simulink model "soc_WLAN_fpga"  (R2024b)
settings: Solver=FixedStepDiscrete  StartTime=0.0  StopTime=stopTime  RelTol=1e-3
PreLoadFcn:
  | addpath(fullfile(matlabroot,'toolbox','whdl','whdlexamples','whdlexamples'));
InitFcn:
  | addpath(fullfile(matlabroot,'toolbox','whdl','whdlexamples','whdlexamples'));
model workspace (MAT data in the model file):
  socvcb = containers.Map
  socvcb.serialization.keys = {}
  socvcb.serialization.values = {}
  socvcb.serialization.uniformity = 0
  socvcb.serialization.keyType = 'double'
  socvcb.serialization.valueType = 'any'
undefined symbols (not defined in the file): Add, bitRatePerOfdmSym, chanBW, coe, cpLen, dataUpsampleFactor, DelayValMaxNsdMinusLastPilotSc, DescramblerInitialSeed, designMultirateFIR, fftLen, filterLatency, filterUpsampleFactor, Fs, Hd, HT_MFMCS0, HT_MFMCS1, HT_MFMCS2, HT_MFMCS3, HT_MFMCS4, HT_MFMCS5, HT_MFMCS6, HT_MFMCS7, HTUnUsedScInd, inputSamplingRate, interp_coeff, maxPilotRefCounterVale, maxPilotsRef, maxPilotsRefNonHT, Ncol_HT, Ncol_NonHT, noDataSubCarriers, Non_HTMCS0, Non_HTMCS1, Non_HTMCS2, Non_HTMCS3, Non_HTMCS4, Non_HTMCS5, Non_HTMCS6, Non_HTMCS7, Nrow_HT, Nrow_NonHT, numDSC_HT, numDSC_HT_vhtSigB, numDSC_NonHT, numDscHT, numDscNonHT, numOfBitsPerOFDMSym, numOfDataBitsPerOFDMSym, numPilots, numScHT, numSCS_HT, numSCS_NonHT, pnSeq, QAM, rxDownsampleFactor, secondPIdx_HT, secondPIdx_NonHT, Shift, VHTMCS0, VHTMCS1 ... (+7)
libraries: hdlsllib x267, simulink x210, dspsigops x22, whdlutilities x10, whdlmod x9, dsphdlfiltering2 x5, dsphdlmathfun2 x4, whdledac x3, hwlogicconnlib x2, commhdlcrc x2, dsphdlsigops2 x2
(part 1 of 14)
settings Model: DataDictionary=wlanhdlRxData.sldd  DataTypeOverride=Off  SimulationMode=accelerator  Creator=The MathWorks, Inc.  LastModifiedBy=wings
settings SolverCC: AlgebraicLoopSolver=TrustRegion  PositivePriorityOrder=on  AutoInsertRateTranBlk=on  MaxZcPerStep=1
settings DataIOCC: SaveTime=off  ReturnWorkspaceOutputs=off
settings OptimizationCC: BlockReduction=off  ConditionallyExecuteInputs=off  DefaultParameterBehavior=Inlined  EnhancedBackFolding=on  PassReuseOutputArgsAs=Individual arguments  ZeroExternalMemoryAtStartup=off  ZeroInternalMemoryAtStartup=off  MaxStackSize=64  OptimizeBlockOrder=speed  DifferentSizesBufferReuse=on  OptimizationCustomize=off  EfficientTunableParamExpr=on
settings DebuggingCC: AlgebraicLoopMsg=error  SingleTaskRateTransMsg=error  IntegerOverflowMsg=none  ParameterPrecisionLossMsg=none  ParameterTunabilityLossMsg=error  UnconnectedInputMsg=warning  UnconnectedOutputMsg=warning  UnconnectedLineMsg=warning  BusObjectLabelMismatch=none  ModelReferenceDataLoggingMessage=none  SubsystemReferenceDiagnosticForUnitTest=warning  SFUnexpectedBacktrackingDiag=warning  SFNoUnconditionalDefaultTransitionDiag=warning  ArithmeticOperatorsInVariantConditions=warning
settings HardwareCC: ProdBitPerPointer=32  ProdBitPerSizeT=32  ProdBitPerPtrDiffT=32  ProdLargestAtomicFloat=None  ProdIntDivRoundTo=Undefined  ProdEndianess=Unspecified  ProdWordSize=32  ProdHWDeviceType=ASIC/FPGA->ASIC/FPGA  TargetBitPerLong=64  TargetBitPerPointer=64  TargetBitPerSizeT=64  TargetBitPerPtrDiffT=64  TargetLongLongMode=on  TargetIntDivRoundTo=Zero  TargetEndianess=LittleEndian  TargetWordSize=64  TargetHWDeviceType=Custom Processor->MATLAB Host Computer  ProdEqTarget=off  HardwareBoardFeatureSet=SoCBlockset
settings ModelReferenceCC: EnableRefExpFcnMdlSchedulingChecks=on  ModelReferenceNumInstancesAllowed=Single
settings SFSimCC: SimUseLocalCustomCode=off
settings RTWCC: Description=Embedded Coder  SystemTargetFile=ert.tlc  HardwareBoard=Xilinx Zynq UltraScale+ RFSoC ZCU111 Evaluation Kit  TLCOptions="-aInlineSetEventsForThisBaseRateFcn=TLC_FALSE -aSuppressMultiTaskScheduler=TLC_FALSE  -aRateBasedStepFcn=0"  TemplateMakefile=ert_default_tmf  GenerateReport=on  RTWUseLocalCustomCode=off  Toolchain=Linaro AArch64 Linux v6.3.1  LaunchReport=on  GPUComputeCapability=3.5  DLArmComputeVersion=19.05
settings CodeAppCC: ForceParamTrailComments=on  IgnoreCustomStorageClasses=off  OperatorAnnotations=on  SimulinkDataObjDesc=on  SFDataObjDesc=on  InsertBlockDesc=on

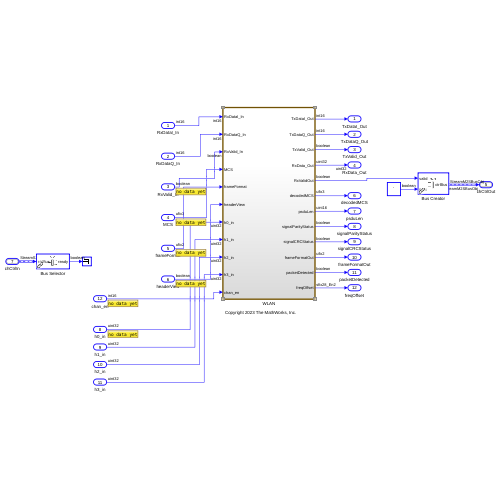
[thumbnail: Simulink's stored preview of the top-level diagram]
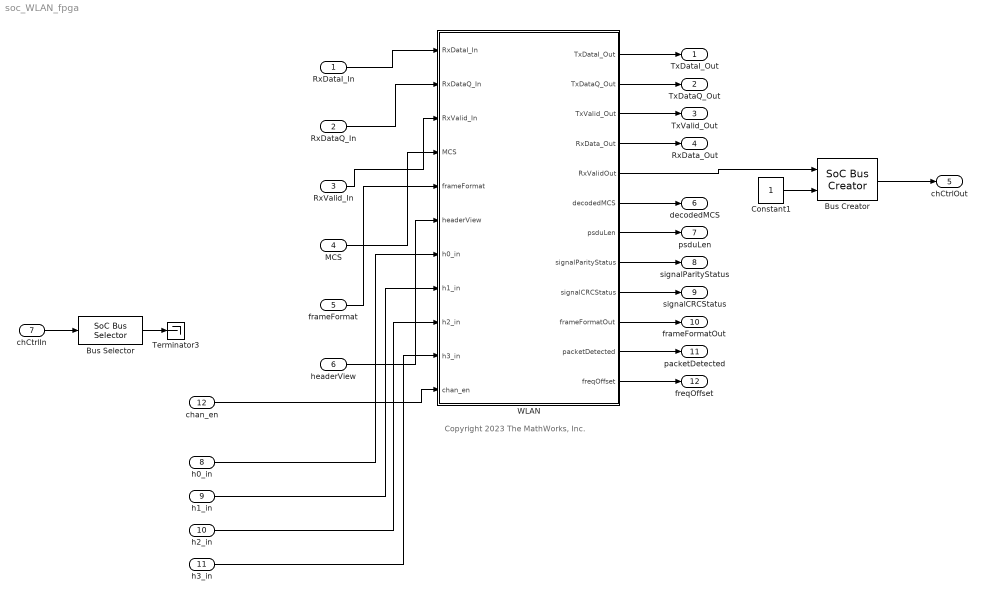
== system soc_WLAN_fpga ==
  note: Copyright 2023 The MathWorks, Inc.
  RxDataI_In : Inport  OutDataTypeStr=int16  PortDimensions=8
  RxDataQ_In : Inport  Port=2  OutDataTypeStr=int16  PortDimensions=8
  RxValid_In : Inport  Port=3  OutDataTypeStr=boolean
  MCS : Inport  Port=4  OutDataTypeStr=fixdt(0,3,0)
  frameFormat : Inport  Port=5  OutDataTypeStr=fixdt(0,2,0)
  headerView : Inport  Port=6  OutDataTypeStr=boolean
  chCtrlIn : Inport  Port=7  OutDataTypeStr=Bus: StreamS2MBusObj  SampleTime=1/inputSamplingRate  BusOutputAsStruct=on
  h0_in : Inport  Port=8  OutDataTypeStr=uint32
  h1_in : Inport  Port=9  OutDataTypeStr=uint32
  h2_in : Inport  Port=10  OutDataTypeStr=uint32
  h3_in : Inport  Port=11  OutDataTypeStr=uint32
  chan_en : Inport  Port=12
  Bus Creator : hwlogicconnlib/SoC Bus Creator  Protocol=Data stream  ctrltype=Valid
  Bus Selector : hwlogicconnlib/SoC Bus Selector  Protocol=Data stream  ctrltype=Ready
  Constant1 : Constant  OutDataTypeStr=boolean  SampleTime=-1
  Terminator3 : Terminator
  WLAN : Subsystem  TreatAsAtomicUnit=on
  TxDataI_Out : Outport
  TxDataQ_Out : Outport  Port=2
  TxValid_Out : Outport  Port=3
  RxData_Out : Outport  Port=4  OutDataTypeStr=uint32
  chCtrlOut : Outport  Port=5  OutDataTypeStr=Bus: StreamM2SBusObj  VectorParamsAs1DForOutWhenUnconnected=off  BusOutputAsStruct=on
  decodedMCS : Outport  Port=6
  psduLen : Outport  Port=7
  signalParityStatus : Outport  Port=8
  signalCRCStatus : Outport  Port=9
  frameFormatOut : Outport  Port=10
  packetDetected : Outport  Port=11
  freqOffset : Outport  Port=12
  wires:
  chCtrlIn/1 -> Bus Selector/1
  Bus Selector/1 -> Terminator3/1
  Bus Creator/1 -> chCtrlOut/1
  Constant1/1 -> Bus Creator/2
  RxDataI_In/1 -> WLAN/1(RxDataI_In)
  RxDataQ_In/1 -> WLAN/2(RxDataQ_In)
  RxValid_In/1 -> WLAN/3(RxValid_In)
  WLAN/1(TxDataI_Out) -> TxDataI_Out/1
  WLAN/2(TxDataQ_Out) -> TxDataQ_Out/1
  WLAN/3(TxValid_Out) -> TxValid_Out/1
  WLAN/4(RxData_Out) -> RxData_Out/1
  WLAN/6(decodedMCS) -> decodedMCS/1
  WLAN/8(signalParityStatus) -> signalParityStatus/1
  WLAN/5(RxValidOut) -> Bus Creator/1
  WLAN/9(signalCRCStatus) -> signalCRCStatus/1
  WLAN/10(frameFormatOut) -> frameFormatOut/1
  WLAN/11(packetDetected) -> packetDetected/1
  WLAN/12(freqOffset) -> freqOffset/1
  MCS/1 -> WLAN/4(MCS)
  frameFormat/1 -> WLAN/5(frameFormat)
  headerView/1 -> WLAN/6(headerView)
  WLAN/7(psduLen) -> psduLen/1
  h1_in/1 -> WLAN/8(h1_in)
  h0_in/1 -> WLAN/7(h0_in)
  h3_in/1 -> WLAN/10(h3_in)
  h2_in/1 -> WLAN/9(h2_in)
  chan_en/1 -> WLAN/11(chan_en)

== system soc_WLAN_fpga/WLAN ==
  RxDataI_In : Inport  OutDataTypeStr=int16
  RxDataQ_In : Inport  Port=2  OutDataTypeStr=int16
  RxValid_In : Inport  Port=3  OutDataTypeStr=boolean
  MCS : Inport  Port=4
  frameFormat : Inport  Port=5
  headerView : Inport  Port=6
  h0_in : Inport  Port=7  OutDataTypeStr=uint32
  h1_in : Inport  Port=8  OutDataTypeStr=uint32
  h2_in : Inport  Port=9  OutDataTypeStr=uint32
  h3_in : Inport  Port=10  OutDataTypeStr=uint32
  chan_en : Inport  Port=11
  Concatention : Subsystem  TreatAsAtomicUnit=on
  Conversion : Subsystem  TreatAsAtomicUnit=on
  Vector Decimator : Subsystem
  Vector Interpolation : Subsystem
  WLAN HDL : Subsystem  TreatAsAtomicUnit=on
  TxDataI_Out : Outport
  TxDataQ_Out : Outport  Port=2
  TxValid_Out : Outport  Port=3
  RxData_Out : Outport  Port=4  OutDataTypeStr=uint32
  RxValidOut : Outport  Port=5
  decodedMCS : Outport  Port=6
  psduLen : Outport  Port=7
  signalParityStatus : Outport  Port=8
  signalCRCStatus : Outport  Port=9
  frameFormatOut : Outport  Port=10
  packetDetected : Outport  Port=11
  freqOffset : Outport  Port=12
  wires:
  Vector Decimator/2(validOut) -> Conversion/2(validIn)
  RxDataQ_In/1 -> Vector Decimator/2(dataQ_in)
  WLAN HDL/9(signalCRCStatus) -> signalCRCStatus/1
  WLAN HDL/5(RxValid_Out) -> RxValidOut/1
  Conversion/2(dataQOut) -> WLAN HDL/2(RxDataQ_In)
  WLAN HDL/3(TxValid_Out) -> Vector Interpolation/3(valid)
  RxValid_In/1 -> Vector Decimator/3(validIn)
  Vector Interpolation/3(txValid) -> TxValid_Out/1
  Conversion/1(dataIOut) -> WLAN HDL/1(RxDataI_In)
  Vector Interpolation/2(txQData) -> TxDataQ_Out/1
  RxDataI_In/1 -> Vector Decimator/1(dataI_in)
  WLAN HDL/10(frameFormatOut) -> frameFormatOut/1
  WLAN HDL/11(packetDetected) -> packetDetected/1
  WLAN HDL/6(decodedMCS) -> decodedMCS/1
  WLAN HDL/4(RxData_Out) -> Concatention/1(dataIn)
  WLAN HDL/1(TxDataI_Out) -> Vector Interpolation/1(dataI_in)
  Vector Interpolation/1(txIData) -> TxDataI_Out/1
  WLAN HDL/8(signalParityStatus) -> signalParityStatus/1
  Conversion/3(validOut) -> WLAN HDL/3(RxValid_In)
  Vector Decimator/1(dataOut) -> Conversion/1(dataIn)
  WLAN HDL/2(TxDataQ_Out) -> Vector Interpolation/2(dataQ_in)
  Concatention/1(dataOut) -> RxData_Out/1
  MCS/1 -> WLAN HDL/4(MCS)
  frameFormat/1 -> WLAN HDL/5(frameFormat)
  headerView/1 -> WLAN HDL/6(headerView)
  WLAN HDL/12(freqOffset) -> freqOffset/1  "freqOffset"
  WLAN HDL/7(psduLen) -> psduLen/1  "decodedPSDULength"
  h1_in/1 -> WLAN HDL/8(h1_in)
  h0_in/1 -> WLAN HDL/7(h0_in)
  h3_in/1 -> WLAN HDL/10(h3_in)
  h2_in/1 -> WLAN HDL/9(h2_in)
  chan_en/1 -> WLAN HDL/11(chan_en)

== system soc_WLAN_fpga/WLAN/Concatention ==
  dataIn : Inport
  Bit Concat : hdlsllib/Logic and Bit Operations/Bit Concat  numInputs=2
  Complex to Real-Imag1 : ComplexToRealImag
  dataOut : Outport
  wires:
  Bit Concat/1 -> dataOut/1
  dataIn/1 -> Complex to Real-Imag1/1
  Complex to Real-Imag1/1 -> Bit Concat/1
  Complex to Real-Imag1/2 -> Bit Concat/2

== system soc_WLAN_fpga/WLAN/Conversion ==
  dataIn : Inport
  validIn : Inport  Port=2
  Complex to Real-Imag : ComplexToRealImag
  Data Type Conversion : DataTypeConversion  OutDataTypeStr=int16  ConvertRealWorld=Stored Integer (SI)  SaturateOnIntegerOverflow=off  RndMeth=Floor
  Data Type Conversion1 : DataTypeConversion  OutDataTypeStr=int16  ConvertRealWorld=Stored Integer (SI)  SaturateOnIntegerOverflow=off  RndMeth=Floor
  dataIOut : Outport
  dataQOut : Outport  Port=2
  validOut : Outport  Port=3
  wires:
  Complex to Real-Imag/1 -> Data Type Conversion/1
  Complex to Real-Imag/2 -> Data Type Conversion1/1
  Data Type Conversion/1 -> dataIOut/1
  dataIn/1 -> Complex to Real-Imag/1
  Data Type Conversion1/1 -> dataQOut/1
  validIn/1 -> validOut/1

== system soc_WLAN_fpga/WLAN/Vector Decimator ==
  dataI_in : Inport
  dataQ_in : Inport  Port=2
  validIn : Inport  Port=3
  Vector Decimation : Subsystem
  dataOut : Outport
  validOut : Outport  Port=2
  wires:
  Vector Decimation/1(dout) -> dataOut/1
  Vector Decimation/2(vout) -> validOut/1
  validIn/1 -> Vector Decimation/3(validIn)
  dataI_in/1 -> Vector Decimation/1(din_real)
  dataQ_in/1 -> Vector Decimation/2(din_img)

== system soc_WLAN_fpga/WLAN/Vector Interpolation ==
  dataI_in : Inport
  dataQ_in : Inport  Port=2
  valid : Inport  Port=3
  Complex to Real-Imag : ComplexToRealImag
  Data Type Conversion : DataTypeConversion  OutDataTypeStr=int16  SaturateOnIntegerOverflow=off  RndMeth=Floor
  Extract Bits : simulink/Logic and Bit Operations/Extract Bits  bitsToExtract=Range starting with most significant bit  numBits=12  bitIdxRange=[0 7]  outScalingMode=Treat bit field as an integer
  Extract Bits1 : simulink/Logic and Bit Operations/Extract Bits  bitsToExtract=Range starting with most significant bit  numBits=12  bitIdxRange=[0 7]  outScalingMode=Treat bit field as an integer
  FIR Interpolator : dsphdlfiltering2/FIR Interpolator  Numerator=interp_coeff  FilterStructure=Direct form systolic  InterpolationFactor=8  NumCycles=1  OptimizeSymmCoeff=off  SimulateUsing=Code generation  roundingMode=Floor  overflowMode=off  CoefficientsDataTypeStr=Inherit: Same word length as input  OutputDataTypeStr=fixdt(1,16,0)  ResetInputPort=off  HDLGlobalReset=off
  Real-Imag to Complex : RealImagToComplex
  Terminator3 : Terminator
  txIData : Outport
  txQData : Outport  Port=2
  txValid : Outport  Port=3
  wires:
  valid/1 -> FIR Interpolator/2
  FIR Interpolator/1 -> Complex to Real-Imag/1
  FIR Interpolator/2 -> txValid/1
  Data Type Conversion/1 -> FIR Interpolator/1
  dataI_in/1 -> Extract Bits/1
  dataQ_in/1 -> Extract Bits1/1
  Real-Imag to Complex/1 -> Data Type Conversion/1
  Extract Bits/1 -> Real-Imag to Complex/1
  Extract Bits1/1 -> Real-Imag to Complex/2
  Complex to Real-Imag/1 -> txIData/1
  Complex to Real-Imag/2 -> txQData/1
  FIR Interpolator/3 -> Terminator3/1

== system soc_WLAN_fpga/WLAN/WLAN HDL ==
  note: Generate Status Signals to monitor Outside FPGA
  note: WLAN Transmit and Receive
  note: Status Signal Generator
  RxDataI_In : Inport
  RxDataQ_In : Inport  Port=2
  RxValid_In : Inport  Port=3
  MCS : Inport  Port=4
  frameFormat : Inport  Port=5
  headerView : Inport  Port=6
  h0_in : Inport  Port=7  OutDataTypeStr=uint32
  h1_in : Inport  Port=8  OutDataTypeStr=uint32
  h2_in : Inport  Port=9  OutDataTypeStr=uint32
  h3_in : Inport  Port=10  OutDataTypeStr=uint32
  chan_en : Inport  Port=11
  Complex to Real-Imag : ComplexToRealImag
  Constellation Formation : Subsystem
  Diagnostic Decoder : Subsystem
  Prepare Inputs : Subsystem
  Prepare Outputs : Subsystem
  Real-Imag to Complex : RealImagToComplex
  WLAN_Tx_Rx : Subsystem
  TxDataI_Out : Outport
  TxDataQ_Out : Outport  Port=2
  TxValid_Out : Outport  Port=3
  RxData_Out : Outport  Port=4
  RxValid_Out : Outport  Port=5
  decodedMCS : Outport  Port=6
  psduLen : Outport  Port=7
  signalParityStatus : Outport  Port=8
  signalCRCStatus : Outport  Port=9
  frameFormatOut : Outport  Port=10
  packetDetected : Outport  Port=11
  freqOffset : Outport  Port=12
  wires:
  WLAN_Tx_Rx/3(diagBus) -> [diagBus]
  WLAN_Tx_Rx/2(txValid) -> Prepare Outputs/2(txvalid)
  WLAN_Tx_Rx/1(txData) -> Prepare Outputs/1(txData)
  Constellation Formation/2(rxValidOut) -> RxValid_Out/1
  Prepare Outputs/2(txValidOut) -> TxValid_Out/1
  Prepare Outputs/1(txDataOut) -> Complex to Real-Imag/1
  headerView/1 -> Constellation Formation/5(hView)
  RxValid_In/1 -> Prepare Inputs/2(rxValid)
  Prepare Inputs/1(rxDataOut) -> WLAN_Tx_Rx/1(rxData)
  Prepare Inputs/2(rxValidOut) -> WLAN_Tx_Rx/2(rxValid)
  Real-Imag to Complex/1 -> Prepare Inputs/1(rxData)
  RxDataI_In/1 -> Real-Imag to Complex/1
  RxDataQ_In/1 -> Real-Imag to Complex/2
  Complex to Real-Imag/1 -> TxDataI_Out/1
  Complex to Real-Imag/2 -> TxDataQ_Out/1
  Constellation Formation/1(rxDataOut) -> RxData_Out/1
  MCS/1 -> WLAN_Tx_Rx/4(MCS)
  frameFormat/1 -> WLAN_Tx_Rx/3(frameFormat)
  [diagBus] -> Diagnostic Decoder/1(diagBus)
  Diagnostic Decoder/1(decodedMCS) -> decodedMCS/1
  Diagnostic Decoder/2(psduLen) -> psduLen/1
  Diagnostic Decoder/3(signalParityStatus) -> signalParityStatus/1
  Diagnostic Decoder/4(signalCRCStatus) -> signalCRCStatus/1
  Diagnostic Decoder/5(frameFormat) -> frameFormatOut/1
  Diagnostic Decoder/6(packetDetected) -> packetDetected/1
  Diagnostic Decoder/7(freqOffset) -> freqOffset/1
  Diagnostic Decoder/8(headerConstellationValid) -> Constellation Formation/1(hValid)
  Diagnostic Decoder/9(headerConstellation) -> Constellation Formation/2(hPoints)
  Diagnostic Decoder/10(dataConstellationValid) -> Constellation Formation/3(dValid)
  Diagnostic Decoder/11(dataConstellation) -> Constellation Formation/4(dPoints)
  h1_in/1 -> WLAN_Tx_Rx/6(h1_in)
  h0_in/1 -> WLAN_Tx_Rx/5(h0_in)
  h3_in/1 -> WLAN_Tx_Rx/8(h3_in)
  h2_in/1 -> WLAN_Tx_Rx/7(h2_in)
  chan_en/1 -> WLAN_Tx_Rx/9(chan_en)

== system soc_WLAN_fpga/WLAN/Vector Decimator/Vector Decimation ==
  din_real : Inport
  din_img : Inport  Port=2
  validIn : Inport  Port=3
  FIR Decimation HDL Optimized : dsphdlfiltering2/FIR Decimator  Numerator=coe  FilterStructure=Direct form systolic  DecimationFactor=8  NumCycles=1  OptimizeSymmCoeff=off  SimulateUsing=Code generation  roundingMode=Floor  overflowMode=off  CoefficientsDataTypeStr=Inherit: Same word length as input  OutputDataTypeStr=fixdt(1,16,0)  ResetInputPort=off  HDLGlobalReset=off
  Real-Imag to Complex : RealImagToComplex
  dout : Outport  VectorParamsAs1DForOutWhenUnconnected=off
  vout : Outport  Port=2  VectorParamsAs1DForOutWhenUnconnected=off
  wires:
  din_real/1 -> Real-Imag to Complex/1  "in2"
  din_img/1 -> Real-Imag to Complex/2  "in2"
  validIn/1 -> FIR Decimation HDL Optimized/2  "in2"
  Real-Imag to Complex/1 -> FIR Decimation HDL Optimized/1  "in2"
  FIR Decimation HDL Optimized/2 -> vout/1
  FIR Decimation HDL Optimized/1 -> dout/1

== system soc_WLAN_fpga/WLAN/WLAN HDL/Constellation Formation ==
  note: NO HDL Block
  note: NO HDL Block
  hValid : Inport
  hPoints : Inport  Port=2
  dValid : Inport  Port=3
  dPoints : Inport  Port=4
  hView : Inport  Port=5
  Data Type Conversion : DataTypeConversion  OutDataTypeStr=int16  ConvertRealWorld=Stored Integer (SI)  SaturateOnIntegerOverflow=off  RndMeth=Floor
  Switch : Switch  Threshold=1  SaturateOnIntegerOverflow=off  InputSameDT=off
  Switch1 : Switch  Threshold=1  SaturateOnIntegerOverflow=off  InputSameDT=off
  Visualize Data Constellation : Subsystem
  Visualize Header Constellation : Subsystem
  rxDataOut : Outport
  rxValidOut : Outport  Port=2
  wires:
  hPoints/1 -> Switch/1, Visualize Header Constellation/1(header constellation points)
  dValid/1 -> Switch1/3, Visualize Data Constellation/Enable
  dPoints/1 -> Switch/3, Visualize Data Constellation/1(data constellation points)
  hValid/1 -> Switch1/1, Visualize Header Constellation/Enable
  Switch/1 -> Data Type Conversion/1
  Switch1/1 -> rxValidOut/1
  hView/1 -> Switch/2, Switch1/2
  Data Type Conversion/1 -> rxDataOut/1

== system soc_WLAN_fpga/WLAN/WLAN HDL/Diagnostic Decoder ==
  diagBus : Inport  OutDataTypeStr=Bus: diagBus
  Bus Selector : BusSelector  OutputSignals=decodedMCS,PSDULen,signalParityStatus,signalCRCStatus,frameFormat,packetDetected,freqOffset,headerConstellation,dataConstellation
  Bus Selector1 : BusSelector  OutputSignals=dataConstellationPoints,dataConstellationValid
  Bus Selector2 : BusSelector  OutputSignals=headerConstellationPoints,headerConstellationValid
  Downsample{,1..10} (11 alike) : DownSample  N=4*chanBW  RateOptions=Allow multirate processing
  Gain : Gain  Gain=wlanConfig.Fs  OutDataTypeStr=fixdt(1,28,2)
  decodedMCS : Outport
  psduLen : Outport  Port=2
  signalParityStatus : Outport  Port=3
  signalCRCStatus : Outport  Port=4
  frameFormat : Outport  Port=5
  packetDetected : Outport  Port=6
  freqOffset : Outport  Port=7
  headerConstellationValid : Outport  Port=8
  headerConstellation : Outport  Port=9
  dataConstellationValid : Outport  Port=10
  dataConstellation : Outport  Port=11
  wires:
  Bus Selector/2 -> Downsample1/1  "<PSDULen>"
  Bus Selector/7 -> Gain/1  "<freqOffset>"
  Gain/1 -> Downsample6/1
  Bus Selector/6 -> Downsample5/1  "<packetDetected>"
  diagBus/1 -> Bus Selector/1
  Bus Selector/1 -> Downsample/1  "<decodedMCS>"
  Bus Selector/3 -> Downsample2/1  "<signalParityStatus>"
  Bus Selector/8 -> Bus Selector2/1  "<headerConstellation>"
  Bus Selector/5 -> Downsample4/1  "<frameFormat>"
  Bus Selector1/2 -> Downsample10/1  "<dataConstellationValid>"
  Bus Selector/4 -> Downsample3/1  "<signalCRCStatus>"
  Bus Selector2/2 -> Downsample8/1  "<headerConstellationValid>"
  Bus Selector1/1 -> Downsample9/1  "<dataConstellationPoints>"
  Bus Selector/9 -> Bus Selector1/1  "<dataConstellation>"
  Bus Selector2/1 -> Downsample7/1  "<headerConstellationPoints>"
  Downsample5/1 -> packetDetected/1
  Downsample/1 -> decodedMCS/1
  Downsample1/1 -> psduLen/1
  Downsample2/1 -> signalParityStatus/1
  Downsample3/1 -> signalCRCStatus/1
  Downsample4/1 -> frameFormat/1
  Downsample6/1 -> freqOffset/1
  Downsample7/1 -> headerConstellation/1
  Downsample8/1 -> headerConstellationValid/1
  Downsample9/1 -> dataConstellation/1
  Downsample10/1 -> dataConstellationValid/1

== system soc_WLAN_fpga/WLAN/WLAN HDL/Prepare Inputs ==
  rxData : Inport
  rxValid : Inport  Port=2
  Bit Shift : hdlsllib/Logic and Bit Operations/Bit Shift  mode=Shift Left Logical  N=4
  Data Type Conversion : DataTypeConversion  OutDataTypeStr=fixdt(1,16,13)  ConvertRealWorld=Stored Integer (SI)  SaturateOnIntegerOverflow=off  RndMeth=Floor
  rxDataOut : Outport
  rxValidOut : Outport  Port=2
  wires:
  Bit Shift/1 -> Data Type Conversion/1
  Data Type Conversion/1 -> rxDataOut/1
  rxValid/1 -> rxValidOut/1
  rxData/1 -> Bit Shift/1

== system soc_WLAN_fpga/WLAN/WLAN HDL/Prepare Outputs ==
  txData : Inport
  txvalid : Inport  Port=2
  Data Type Conversion : DataTypeConversion  OutDataTypeStr=int16  ConvertRealWorld=Stored Integer (SI)  SaturateOnIntegerOverflow=off  RndMeth=Floor
  txDataOut : Outport
  txValidOut : Outport  Port=2
  wires:
  txData/1 -> Data Type Conversion/1
  txvalid/1 -> txValidOut/1
  Data Type Conversion/1 -> txDataOut/1

== system soc_WLAN_fpga/WLAN/WLAN HDL/WLAN_Tx_Rx ==
  rxData : Inport
  rxValid : Inport  Port=2
  frameFormat : Inport  Port=3
  MCS : Inport  Port=4
  h0_in : Inport  Port=5  OutDataTypeStr=uint32
  h1_in : Inport  Port=6  OutDataTypeStr=uint32
  h2_in : Inport  Port=7  OutDataTypeStr=uint32
  h3_in : Inport  Port=8  OutDataTypeStr=uint32
  chan_en : Inport  Port=9  OutDataTypeStr=int16
  4-tap FIR Filter : Subsystem
  Data Type Conversion : DataTypeConversion  OutDataTypeStr=fixdt(0,2,0)  ConvertRealWorld=Stored Integer (SI)  SaturateOnIntegerOverflow=off  RndMeth=Floor
  Data Type Conversion1 : DataTypeConversion  OutDataTypeStr=fixdt(0,3,0)  ConvertRealWorld=Stored Integer (SI)  SaturateOnIntegerOverflow=off  RndMeth=Floor
  Decimator : Subsystem  Variant=on
  Delay{1,4,7,10..11} (5 alike) : Delay  DelayLength=1  InitialCondition=0
  Downsample : DownSample  N=rxDownsampleFactor  RateOptions=Allow multirate processing
  Downsample1 : DownSample  N=rxDownsampleFactor  RateOptions=Allow multirate processing
  Switch : Switch  Criteria=u2 > Threshold  SaturateOnIntegerOverflow=off  InputSameDT=off
  WLAN_Rx : Subsystem
  WLAN_Tx : Subsystem  Variant=on
  txData : Outport
  txValid : Outport  Port=2
  diagBus : Outport  Port=3
  wires:
  MCS/1 -> Data Type Conversion1/1
  frameFormat/1 -> Data Type Conversion/1
  WLAN_Tx/1(txData) -> txData/1
  WLAN_Rx/1(diagBus) -> diagBus/1
  WLAN_Tx/2(txValid) -> txValid/1
  Data Type Conversion/1 -> WLAN_Tx/1(frameFormat)
  Data Type Conversion1/1 -> WLAN_Tx/2(MCS)
  Downsample/1 -> WLAN_Rx/1(dataIn)
  Downsample1/1 -> WLAN_Rx/2(validIn)
  rxData/1 -> Decimator/1(rxDataIn)
  rxValid/1 -> Decimator/2(rxValidIn)
  Decimator/2(rxValidOut) -> Downsample1/1
  h1_in/1 -> Delay7/1
  h0_in/1 -> Delay4/1
  Delay11/1 -> 4-tap FIR Filter/5(h3_in)
  h2_in/1 -> Delay10/1
  h3_in/1 -> Delay11/1
  Delay4/1 -> 4-tap FIR Filter/2(h0_in)
  Delay7/1 -> 4-tap FIR Filter/3(h1_in)
  Delay10/1 -> 4-tap FIR Filter/4(h2_in)
  4-tap FIR Filter/1(data_out) -> Switch/1
  chan_en/1 -> Delay1/1
  Delay1/1 -> Switch/2
  Decimator/1(rxDataOut) -> 4-tap FIR Filter/1(data_in), Switch/3
  Switch/1 -> Downsample/1

== system soc_WLAN_fpga/WLAN/WLAN HDL/Constellation Formation/Visualize Data Constellation ==
  data constellation points : Inport
  Enable : EnablePort
  Data Constellation Diagram : ConstellationDiagram  WindowPosition=[462.000000,49.000000,431.000000,398.000000,]  ScopeFrameLocation=window  SymbolsToDisplaySource=Property  SymbolsToDisplay=1e7  ReferenceConstellation="[0.70711+0.70711i        -0.70711+0.70711i        -0.70711-0.70711i         0.70711-0.70711i]"  Title=Data Constellation  XLimits=[-1.3903 1.3913]  YLimits=[-1.3903 1.3913]  DefaultConfigurationName=comm.scopes.ConstellationDiagramBlockCfg
  wires:
  data constellation points/1 -> Data Constellation Diagram/1

== system soc_WLAN_fpga/WLAN/WLAN HDL/Constellation Formation/Visualize Header Constellation ==
  header constellation points : Inport
  Enable : EnablePort
  Header Constellation Diagram : ConstellationDiagram  WindowPosition=[462.000000,49.000000,431.000000,398.000000,]  ScopeFrameLocation=window  SymbolsToDisplaySource=Property  SymbolsToDisplay=1e6  ReferenceConstellation="[1+0i           -1+1.2246e-16i]"  Title=Header Constellation  XLimits=[-1.0442 1.0248]  YLimits=[-1.0442 1.0248]  DefaultConfigurationName=comm.scopes.ConstellationDiagramBlockCfg
  wires:
  header constellation points/1 -> Header Constellation Diagram/1

== system soc_WLAN_fpga/WLAN/WLAN HDL/WLAN_Tx_Rx/4-tap FIR Filter ==
  data_in : Inport
  h0_in : Inport  Port=2  OutDataTypeStr=uint32
  h1_in : Inport  Port=3  OutDataTypeStr=uint32
  h2_in : Inport  Port=4  OutDataTypeStr=uint32
  h3_in : Inport  Port=5  OutDataTypeStr=uint32
  32-bit Packed Complex TO sfix Complex : Subsystem
  32-bit Packed Complex TO sfix Complex1 : Subsystem
  32-bit Packed Complex TO sfix Complex2 : Subsystem
  32-bit Packed Complex TO sfix Complex3 : Subsystem
  Data Type Conversion{1..5} (5 alike) : DataTypeConversion  OutDataTypeStr=fixdt(1,16,13)  SaturateOnIntegerOverflow=off  RndMeth=Floor
  Delay : Delay  DelayLength=1
  Delay1 : Delay  DelayLength=1
  Delay2 : Delay  DelayLength=1
  Product{,1..3} (4 alike) : Product
  Sum : Sum  Inputs=|++++
  data_out : Outport
  wires:
  data_in/1 -> Delay/1, Product/1
  Delay/1 -> Delay1/1, Product1/1
  Delay1/1 -> Delay2/1, Product2/1
  32-bit Packed Complex TO sfix Complex2/1(c) -> Product2/2
  32-bit Packed Complex TO sfix Complex1/1(c) -> Product1/2
  32-bit Packed Complex TO sfix Complex3/1(c) -> Product3/2
  Product/1 -> Data Type Conversion4/1
  Product1/1 -> Data Type Conversion3/1
  Product2/1 -> Data Type Conversion2/1
  Product3/1 -> Data Type Conversion1/1
  Sum/1 -> Data Type Conversion5/1
  Delay2/1 -> Product3/1
  Data Type Conversion1/1 -> Sum/1
  Data Type Conversion2/1 -> Sum/2
  Data Type Conversion3/1 -> Sum/3
  Data Type Conversion4/1 -> Sum/4
  Data Type Conversion5/1 -> data_out/1
  32-bit Packed Complex TO sfix Complex/1(c) -> Product/2
  h0_in/1 -> 32-bit Packed Complex TO sfix Complex/1(i)
  h3_in/1 -> 32-bit Packed Complex TO sfix Complex3/1(i)
  h2_in/1 -> 32-bit Packed Complex TO sfix Complex2/1(i)
  h1_in/1 -> 32-bit Packed Complex TO sfix Complex1/1(i)

== system soc_WLAN_fpga/WLAN/WLAN HDL/WLAN_Tx_Rx/Decimator ==
  note: 1) Add Subsystem or Model blocks as valid variant choices.
      | 2) You cannot connect blocks at this level. At simulation, connectivity is automatically
      | determined, based on the active variant and port name matching.
  rxDataIn : Inport
  rxValidIn : Inport  Port=2
  Decimate_20MHz : Subsystem  VariantControl=chanBW == 1
  Decimate_40MHz : Subsystem  VariantControl=chanBW == 2
  rxDataOut : Outport
  rxValidOut : Outport  Port=2

== system soc_WLAN_fpga/WLAN/WLAN HDL/WLAN_Tx_Rx/WLAN_Rx ==
  dataIn : Inport
  validIn : Inport  Port=2
  Constant : Constant  Value=false  SampleTime=1/wlanConfig.Fs
  Terminator : Terminator
  Terminator1 : Terminator
  WLANHDLReceiver : Subsystem
  diagBus : Outport
  wires:
  dataIn/1 -> WLANHDLReceiver/1(dataIn)
  validIn/1 -> WLANHDLReceiver/2(validIn)
  Constant/1 -> WLANHDLReceiver/3(startIn)
  WLANHDLReceiver/1(rxBits) -> Terminator/1
  WLANHDLReceiver/2(validOut) -> Terminator1/1
  WLANHDLReceiver/3(diagBus) -> diagBus/1

== system soc_WLAN_fpga/WLAN/WLAN HDL/WLAN_Tx_Rx/WLAN_Tx ==
  note: 1) Add Subsystem or Model blocks as valid variant choices.
      | 2) You cannot connect blocks at this level. At simulation, connectivity is automatically
      | determined, based on the active variant and port name matching.
  frameFormat : Inport
  MCS : Inport  Port=2
  WLAN_Tx_20MHz : Subsystem  VariantControl=chanBW == 1
  WLAN_Tx_40MHz : Subsystem  VariantControl=chanBW == 2
  txData : Outport
  txValid : Outport  Port=2

== system soc_WLAN_fpga/WLAN/WLAN HDL/WLAN_Tx_Rx/4-tap FIR Filter/32-bit Packed Complex TO sfix Complex ==
  i : Inport
  Bit Slice : hdlsllib/Logic and Bit Operations/Bit Slice  lidx=31  ridx=16
  Bit Slice1 : hdlsllib/Logic and Bit Operations/Bit Slice  lidx=15  ridx=0
  Data Type Conversion6 : DataTypeConversion  OutDataTypeStr=fixdt(1,16,13)  ConvertRealWorld=Stored Integer (SI)  SaturateOnIntegerOverflow=off  RndMeth=Floor
  Data Type Conversion7 : DataTypeConversion  OutDataTypeStr=fixdt(1,16,13)  ConvertRealWorld=Stored Integer (SI)  SaturateOnIntegerOverflow=off  RndMeth=Floor
  Real-Imag to Complex : RealImagToComplex
  c : Outport
  wires:
  Bit Slice1/1 -> Data Type Conversion7/1
  Data Type Conversion7/1 -> Real-Imag to Complex/2
  Data Type Conversion6/1 -> Real-Imag to Complex/1
  Bit Slice/1 -> Data Type Conversion6/1
  Real-Imag to Complex/1 -> c/1
  i/1 -> Bit Slice1/1, Bit Slice/1

== system soc_WLAN_fpga/WLAN/WLAN HDL/WLAN_Tx_Rx/4-tap FIR Filter/32-bit Packed Complex TO sfix Complex1 ==
  i : Inport
  Bit Slice : hdlsllib/Logic and Bit Operations/Bit Slice  lidx=31  ridx=16
  Bit Slice1 : hdlsllib/Logic and Bit Operations/Bit Slice  lidx=15  ridx=0
  Data Type Conversion6 : DataTypeConversion  OutDataTypeStr=fixdt(1,16,13)  ConvertRealWorld=Stored Integer (SI)  SaturateOnIntegerOverflow=off  RndMeth=Floor
  Data Type Conversion7 : DataTypeConversion  OutDataTypeStr=fixdt(1,16,13)  ConvertRealWorld=Stored Integer (SI)  SaturateOnIntegerOverflow=off  RndMeth=Floor
  Real-Imag to Complex : RealImagToComplex
  c : Outport
  wires:
  i/1 -> Bit Slice/1, Bit Slice1/1
  Real-Imag to Complex/1 -> c/1
  Bit Slice/1 -> Data Type Conversion6/1
  Data Type Conversion6/1 -> Real-Imag to Complex/1
  Data Type Conversion7/1 -> Real-Imag to Complex/2
  Bit Slice1/1 -> Data Type Conversion7/1

== system soc_WLAN_fpga/WLAN/WLAN HDL/WLAN_Tx_Rx/4-tap FIR Filter/32-bit Packed Complex TO sfix Complex2 ==
  i : Inport
  Bit Slice : hdlsllib/Logic and Bit Operations/Bit Slice  lidx=31  ridx=16
  Bit Slice1 : hdlsllib/Logic and Bit Operations/Bit Slice  lidx=15  ridx=0
  Data Type Conversion6 : DataTypeConversion  OutDataTypeStr=fixdt(1,16,13)  ConvertRealWorld=Stored Integer (SI)  SaturateOnIntegerOverflow=off  RndMeth=Floor
  Data Type Conversion7 : DataTypeConversion  OutDataTypeStr=fixdt(1,16,13)  ConvertRealWorld=Stored Integer (SI)  SaturateOnIntegerOverflow=off  RndMeth=Floor
  Real-Imag to Complex : RealImagToComplex
  c : Outport
  wires:
  Bit Slice1/1 -> Data Type Conversion7/1
  Data Type Conversion7/1 -> Real-Imag to Complex/2
  Data Type Conversion6/1 -> Real-Imag to Complex/1
  Bit Slice/1 -> Data Type Conversion6/1
  Real-Imag to Complex/1 -> c/1
  i/1 -> Bit Slice1/1, Bit Slice/1

== system soc_WLAN_fpga/WLAN/WLAN HDL/WLAN_Tx_Rx/4-tap FIR Filter/32-bit Packed Complex TO sfix Complex3 ==
  i : Inport
  Bit Slice : hdlsllib/Logic and Bit Operations/Bit Slice  lidx=31  ridx=16
  Bit Slice1 : hdlsllib/Logic and Bit Operations/Bit Slice  lidx=15  ridx=0
  Data Type Conversion6 : DataTypeConversion  OutDataTypeStr=fixdt(1,16,13)  ConvertRealWorld=Stored Integer (SI)  SaturateOnIntegerOverflow=off  RndMeth=Floor
  Data Type Conversion7 : DataTypeConversion  OutDataTypeStr=fixdt(1,16,13)  ConvertRealWorld=Stored Integer (SI)  SaturateOnIntegerOverflow=off  RndMeth=Floor
  Real-Imag to Complex : RealImagToComplex
  c : Outport
  wires:
  i/1 -> Bit Slice/1, Bit Slice1/1
  Real-Imag to Complex/1 -> c/1
  Bit Slice/1 -> Data Type Conversion6/1
  Data Type Conversion6/1 -> Real-Imag to Complex/1
  Data Type Conversion7/1 -> Real-Imag to Complex/2
  Bit Slice1/1 -> Data Type Conversion7/1

== system soc_WLAN_fpga/WLAN/WLAN HDL/WLAN_Tx_Rx/Decimator/Decimate_20MHz ==
  rxDataIn : Inport
  rxValidIn : Inport  Port=2
  FIR Decimator : dsphdlfiltering2/FIR Decimator  Numerator=designMultirateFIR(1,2)  FilterStructure=Direct form systolic  DecimationFactor=2  NumCycles=1  OptimizeSymmCoeff=off  SimulateUsing=Code generation  roundingMode=Floor  overflowMode=off  CoefficientsDataTypeStr=Inherit: Same word length as input  OutputDataTypeStr=fixdt(1,16,13)  ResetInputPort=off  HDLGlobalReset=off
  rxDataOut : Outport
  rxValidOut : Outport  Port=2
  wires:
  rxDataIn/1 -> FIR Decimator/1
  rxValidIn/1 -> FIR Decimator/2
  FIR Decimator/1 -> rxDataOut/1
  FIR Decimator/2 -> rxValidOut/1

== system soc_WLAN_fpga/WLAN/WLAN HDL/WLAN_Tx_Rx/Decimator/Decimate_40MHz ==
  rxDataIn : Inport
  rxValidIn : Inport  Port=2
  rxDataOut : Outport
  rxValidOut : Outport  Port=2
  wires:
  rxDataIn/1 -> rxDataOut/1
  rxValidIn/1 -> rxValidOut/1

== system soc_WLAN_fpga/WLAN/WLAN HDL/WLAN_Tx_Rx/WLAN_Rx/WLANHDLReceiver ==
  dataIn : Inport
  validIn : Inport  Port=2
  startIn : Inport  Port=3
  Bus Creator : BusCreator  Inputs=9  OutDataTypeStr=Bus: diagBus  NonVirtualBus=on
  DataRecovery : Subsystem
      settings: PortSchema="{\"entries\":[{\"content\":{\"sides\":[{\"content\":{\"connectorIds\":[\"In1\",\"In2\",\"In3\",\"In4\"]},\"type\":\"ConnectorPlacement.EquallySpacedRectSide\",\"uuid\":\"b7cf2579-28ec-4816-83df-12e2b491458b\"},{\"content\":{\"connectorIds\":[\"Out1\",\"Out2\",\"Out3\",\"Out4\",\"Out5\",\"Out6\",\"Out7\"],\"side\":\"RIGHT\"},\"type\":\"ConnectorPlacement.EquallySpacedRectSide\",\"uuid\":\"fa0e2968-ac95-40d1-8a27-544e39e82f01\"},{\"content\":{\"connectorIds\":[\"In5\",\"In6\",\"In7\",\"In8\"],\"side\":\"TOP\"},\"type\":\"ConnectorPlacement.EquallySpacedRectSide\",\"uuid\":\"f64cbe73-7fb9-4770-b375-6943a3df00a9\"},{\"content\":{\"side\":\"BOTTOM\"},\"type\":\"ConnectorPlacement.EquallySpacedRectSide\",\"uuid\":\"0adee36d-ccc0-446a-b50c-46b53e24ab60\"}]},\"type\":\"ConnectorPlacement.EquallySpacedConnector\",\"uuid\":\"0e8699ac-b090-41df-92aa-01d6c74be23a\"}],\"packageUris\":[\"http://schema.mathworks.com/mf0/Connector/R2020b\"],\"version\":\"1.0\"}"
  Delay{,1..4,9..10,12,14..15} (10 alike) : Delay  DelayLength=1
  Delay{5..8,11} (5 alike) : Delay  DelayLength=4
  FrameFormatController : Subsystem
  FrameFormatDetectionAndSignalRecovery : Subsystem
  HT_VHTCPEEstAndCorrection : Subsystem
  HT_VHTChannelEstAndEqualize : Subsystem
      settings: PortSchema="{\"entries\":[{\"content\":{\"sides\":[{\"content\":{\"connectorIds\":[\"In1\",\"In2\",\"In3\",\"In4\"]},\"type\":\"ConnectorPlacement.EquallySpacedRectSide\",\"uuid\":\"1f8073a4-ed91-4f6e-9302-7b0a33bf6f97\"},{\"content\":{\"connectorIds\":[\"Out1\",\"Out2\",\"Out3\",\"Out4\",\"Out5\"],\"side\":\"RIGHT\"},\"type\":\"ConnectorPlacement.EquallySpacedRectSide\",\"uuid\":\"1daa546e-41f4-446b-a326-9a35439a4956\"},{\"content\":{\"connectorIds\":[\"In5\",\"In6\"],\"side\":\"TOP\"},\"type\":\"ConnectorPlacement.EquallySpacedRectSide\",\"uuid\":\"b2fabb3e-3c28-45a1-838f-39a04fb79cd0\"}]},\"type\":\"ConnectorPlacement.EquallySpacedConnector\",\"uuid\":\"1b44fe4e-3b1a-4915-bf44-7650a2b995e5\"}],\"packageUris\":[\"http://schema.mathworks.com/mf0/Connector/R2020b\"],\"version\":\"1.0\"}"
  NonHTCPEEstAndCorrection : Subsystem
  NonHTChannelEstAndEqualize : Subsystem
  OFDMDemodulation : Subsystem
  WLANTimeAndFrequencySynchronization : Subsystem
  diagBusControl : Subsystem
  rxBits : Outport
  validOut : Outport  Port=2
  diagBus : Outport  Port=3
  wires:
  HT_VHTCPEEstAndCorrection/3(rstOut) -> FrameFormatController/8(HTRst)
  NonHTChannelEstAndEqualize/1(dataOut) -> NonHTCPEEstAndCorrection/1(dataIn)
  HT_VHTChannelEstAndEqualize/5(rstOut) -> HT_VHTCPEEstAndCorrection/5(rstIn)
  WLANTimeAndFrequencySynchronization/3(rstOut) -> OFDMDemodulation/3(rstIn)
  HT_VHTChannelEstAndEqualize/4(formatOut) -> HT_VHTCPEEstAndCorrection/4(formatDetected)
  OFDMDemodulation/5(rstOut) -> NonHTChannelEstAndEqualize/5(rstIn), Delay11/1
  Delay9/1 -> FrameFormatController/1(NonHTDataIn)
  HT_VHTChannelEstAndEqualize/2(validOut) -> HT_VHTCPEEstAndCorrection/2(validIn)
  HT_VHTChannelEstAndEqualize/1(dataOut) -> HT_VHTCPEEstAndCorrection/1(dataIn)
  WLANTimeAndFrequencySynchronization/2(validOut) -> OFDMDemodulation/2(validIn)
  Delay15/1 -> FrameFormatController/4(NonHTRst)
  FrameFormatController/3(numSCs) -> DataRecovery/3(numSCs)
  Delay10/1 -> FrameFormatController/2(NonHTValid)
  Delay14/1 -> FrameFormatController/3(numSymb)
  NonHTChannelEstAndEqualize/3(symbNumOut) -> NonHTCPEEstAndCorrection/3(symbNum)
  startIn/1 -> WLANTimeAndFrequencySynchronization/3(startIn)
  FrameFormatController/1(dataOut) -> DataRecovery/1(dataIn)
  FrameFormatController/4(rstOut) -> DataRecovery/4(rstIn)
  Delay6/1 -> HT_VHTChannelEstAndEqualize/2(validIn)
  FrameFormatController/2(validOut) -> DataRecovery/2(validIn)
  FrameFormatDetectionAndSignalRecovery/2(CRCCheck) -> Delay1/1
  Delay3/1 -> DataRecovery/8(psduLen)
  DataRecovery/6(dataBits) -> rxBits/1
  Delay/1 -> DataRecovery/7(MCS), diagBusControl/1(MCS)
  OFDMDemodulation/4(symbRst) -> NonHTChannelEstAndEqualize/4(symbRst), Delay8/1
  Delay8/1 -> HT_VHTChannelEstAndEqualize/4(symbRst)
  FrameFormatDetectionAndSignalRecovery/5(HTCRCStatus) -> Delay4/1
  validIn/1 -> WLANTimeAndFrequencySynchronization/2(validIn)
  Bus Creator/1 -> diagBus/1
  dataIn/1 -> WLANTimeAndFrequencySynchronization/1(dataIn)
  Delay5/1 -> HT_VHTChannelEstAndEqualize/1(dataIn)
  NonHTCPEEstAndCorrection/2(validOut) -> FrameFormatDetectionAndSignalRecovery/2(validIn), Delay10/1
  NonHTChannelEstAndEqualize/2(validOut) -> NonHTCPEEstAndCorrection/2(sampleIn)
  HT_VHTCPEEstAndCorrection/1(dataOut) -> FrameFormatController/6(HTDataIn)
  WLANTimeAndFrequencySynchronization/1(dataOut) -> OFDMDemodulation/1(dataIn)
  HT_VHTChannelEstAndEqualize/3(vhtSigBVld) -> HT_VHTCPEEstAndCorrection/3(vhtSigB)
  Delay7/1 -> HT_VHTChannelEstAndEqualize/3(symbNum)
  OFDMDemodulation/2(validOut) -> NonHTChannelEstAndEqualize/2(validIn), Delay6/1
  NonHTCPEEstAndCorrection/4(rstOut) -> FrameFormatDetectionAndSignalRecovery/4(rstIn), Delay15/1
  HT_VHTCPEEstAndCorrection/2(validOut) -> FrameFormatController/7(HTValid)
  FrameFormatDetectionAndSignalRecovery/3(frameFormat) -> Delay2/1
  DataRecovery/7(validOut) -> validOut/1
  NonHTCPEEstAndCorrection/1(dataOut) -> FrameFormatDetectionAndSignalRecovery/1(dataIn), Delay9/1
  Delay2/1 -> FrameFormatController/5(formatDetected), HT_VHTChannelEstAndEqualize/6(formatIn), DataRecovery/5(frameFormat), diagBusControl/3(frameFormatIn)
  NonHTCPEEstAndCorrection/3(symbNumOut) -> FrameFormatDetectionAndSignalRecovery/3(symbNum), Delay14/1
  NonHTChannelEstAndEqualize/4(rstOut) -> NonHTCPEEstAndCorrection/4(rstIn)
  OFDMDemodulation/1(dataOut) -> NonHTChannelEstAndEqualize/1(dataIn), Delay5/1
  FrameFormatDetectionAndSignalRecovery/1(decodedMCS) -> Delay/1
  FrameFormatDetectionAndSignalRecovery/4(PSDULength) -> Delay3/1
  OFDMDemodulation/3("symbNum ") -> NonHTChannelEstAndEqualize/3(symbNum), Delay7/1
  Delay11/1 -> diagBusControl/6(packetOut), HT_VHTChannelEstAndEqualize/5(rstIn)
  FrameFormatDetectionAndSignalRecovery/7(numOFDMSymbVHT) -> Delay12/1
  Delay12/1 -> DataRecovery/6(numOFDMSymbVHT)
  diagBusControl/1(decodedMCS) -> Bus Creator/1  "decodedMCS"
  diagBusControl/2(psduLen) -> Bus Creator/2  "PSDULen"
  diagBusControl/3(signalParityStatus) -> Bus Creator/3  "signalParityStatus"
  diagBusControl/4(signalCRCStatus) -> Bus Creator/4  "signalCRCStatus"
  diagBusControl/5(frameFormat) -> Bus Creator/5  "frameFormat"
  diagBusControl/6(headerConstellation) -> Bus Creator/6  "headerConstellation"
  diagBusControl/7(dataConstellation) -> Bus Creator/7  "dataConstellation"
  diagBusControl/8(packetDetected) -> Bus Creator/8  "packetDetected"
  diagBusControl/9(freqOffset) -> Bus Creator/9  "freqOffset"
  Delay1/1 -> diagBusControl/2(signalParity)
  Delay4/1 -> diagBusControl/4(HTSigCRCCheck)
  FrameFormatDetectionAndSignalRecovery/6(headerConstellation) -> diagBusControl/5(headerConst)  "headerConstellation"
  WLANTimeAndFrequencySynchronization/4(freqOffset) -> diagBusControl/7(freqOff)
  DataRecovery/2(VHTSigBCRCStatus) -> diagBusControl/9("VHTSigCRCCheck ")
  DataRecovery/1(psduLenOut) -> diagBusControl/8(psduLength)  "PSDULenOut"
  DataRecovery/3(dataConstellation) -> diagBusControl/10(dataConst)  "dataConstellation"
  DataRecovery/4(dataConstellationValid) -> diagBusControl/11(dataConstValid)
  DataRecovery/5(rstOut) -> diagBusControl/12(rst)

== system soc_WLAN_fpga/WLAN/WLAN HDL/WLAN_Tx_Rx/WLAN_Tx/WLAN_Tx_20MHz ==
  note: LUT Index is selected based on Frame Format and MCS
  frameFormat : Inport
  MCS : Inport  Port=2
  Constant : Constant  Value=true  SampleTime=1/inputSamplingRate
  Constant1 : Constant  Value=0  OutDataTypeStr=fixdt(0,5,0)  SampleTime=1/inputSamplingRate
  Constant10 : Constant  Value=18  OutDataTypeStr=fixdt(0,5,0)  SampleTime=1/inputSamplingRate
  Constant11 : Constant  Value=4  OutDataTypeStr=fixdt(0,5,0)  SampleTime=1/inputSamplingRate
  Constant12 : Constant  Value=5  OutDataTypeStr=fixdt(0,5,0)  SampleTime=1/inputSamplingRate
  Constant13 : Constant  Value=6  OutDataTypeStr=fixdt(0,5,0)  SampleTime=1/inputSamplingRate
  Constant14 : Constant  Value=7  OutDataTypeStr=fixdt(0,5,0)  SampleTime=1/inputSamplingRate
  Constant15 : Constant  Value=11  OutDataTypeStr=fixdt(0,5,0)  SampleTime=1/inputSamplingRate
  Constant16 : Constant  Value=12  OutDataTypeStr=fixdt(0,5,0)  SampleTime=1/inputSamplingRate
  Constant17 : Constant  Value=13  OutDataTypeStr=fixdt(0,5,0)  SampleTime=1/inputSamplingRate
  Constant18 : Constant  Value=14  OutDataTypeStr=fixdt(0,5,0)  SampleTime=1/inputSamplingRate
  Constant19 : Constant  Value=15  OutDataTypeStr=fixdt(0,5,0)  SampleTime=1/inputSamplingRate
  Constant2 : Constant  OutDataTypeStr=fixdt(0,5,0)  SampleTime=1/inputSamplingRate
  Constant20 : Constant  Value=19  OutDataTypeStr=fixdt(0,5,0)  SampleTime=1/inputSamplingRate
  Constant21 : Constant  Value=20  OutDataTypeStr=fixdt(0,5,0)  SampleTime=1/inputSamplingRate
  Constant22 : Constant  Value=21  OutDataTypeStr=fixdt(0,5,0)  SampleTime=1/inputSamplingRate
  Constant23 : Constant  Value=22  OutDataTypeStr=fixdt(0,5,0)  SampleTime=1/inputSamplingRate
  Constant24 : Constant  Value=23  OutDataTypeStr=fixdt(0,5,0)  SampleTime=1/inputSamplingRate
  Constant3 : Constant  Value=2  OutDataTypeStr=fixdt(0,5,0)  SampleTime=1/inputSamplingRate
  Constant4 : Constant  Value=3  OutDataTypeStr=fixdt(0,5,0)  SampleTime=1/inputSamplingRate
  Constant5 : Constant  Value=8  OutDataTypeStr=fixdt(0,5,0)  SampleTime=1/inputSamplingRate
  Constant6 : Constant  Value=9  OutDataTypeStr=fixdt(0,5,0)  SampleTime=1/inputSamplingRate
  Constant7 : Constant  Value=10  OutDataTypeStr=fixdt(0,5,0)  SampleTime=1/inputSamplingRate
  Constant8 : Constant  Value=16  OutDataTypeStr=fixdt(0,5,0)  SampleTime=1/inputSamplingRate
  Constant9 : Constant  Value=17  OutDataTypeStr=fixdt(0,5,0)  SampleTime=1/inputSamplingRate
  Delay : Delay
  Multiport Switch : MultiPortSwitch  DataPortOrder=Zero-based contiguous  Inputs=8  zeroidx=on  SaturateOnIntegerOverflow=off  InputSameDT=off
  Multiport Switch1 : MultiPortSwitch  DataPortOrder=Zero-based contiguous  DataPortIndices={0,1,2,3,8,9,10,16,17,18}  zeroidx=on  SaturateOnIntegerOverflow=off  InputSameDT=off
  Multiport Switch2 : MultiPortSwitch  DataPortOrder=Zero-based contiguous  Inputs=8  DataPortIndices={8,9,10}  zeroidx=on  SaturateOnIntegerOverflow=off  InputSameDT=off
  Multiport Switch3 : MultiPortSwitch  DataPortOrder=Zero-based contiguous  Inputs=8  DataPortIndices={16,17,18}  zeroidx=on  SaturateOnIntegerOverflow=off  InputSameDT=off
  Tx_LUT_Selection : Subsystem
  txData : Outport
  txValid : Outport  Port=2
  wires:
  Multiport Switch1/1 -> Tx_LUT_Selection/1(LUTSelect)
  Constant1/1 -> Multiport Switch/2
  Constant/1 -> Delay/1
  Constant3/1 -> Multiport Switch/4
  Constant5/1 -> Multiport Switch2/2
  Constant4/1 -> Multiport Switch/5
  Constant9/1 -> Multiport Switch3/3
  Constant6/1 -> Multiport Switch2/3
  Constant8/1 -> Multiport Switch3/2
  Multiport Switch/1 -> Multiport Switch1/2
  MCS/1 -> Multiport Switch3/1, Multiport Switch/1, Multiport Switch2/1
  Constant2/1 -> Multiport Switch/3
  Constant7/1 -> Multiport Switch2/4
  Constant10/1 -> Multiport Switch3/4
  Tx_LUT_Selection/1(txData) -> txData/1
  Multiport Switch3/1 -> Multiport Switch1/4
  frameFormat/1 -> Multiport Switch1/1
  Multiport Switch2/1 -> Multiport Switch1/3
  Delay/1 -> txValid/1
  Constant11/1 -> Multiport Switch/6
  Constant12/1 -> Multiport Switch/7
  Constant13/1 -> Multiport Switch/8
  Constant14/1 -> Multiport Switch/9
  Constant15/1 -> Multiport Switch2/5
  Constant16/1 -> Multiport Switch2/6
  Constant17/1 -> Multiport Switch2/7
  Constant18/1 -> Multiport Switch2/8
  Constant19/1 -> Multiport Switch2/9
  Constant20/1 -> Multiport Switch3/5
  Constant21/1 -> Multiport Switch3/6
  Constant22/1 -> Multiport Switch3/7
  Constant23/1 -> Multiport Switch3/8
  Constant24/1 -> Multiport Switch3/9

== system soc_WLAN_fpga/WLAN/WLAN HDL/WLAN_Tx_Rx/WLAN_Tx/WLAN_Tx_40MHz ==
  note: LUT Index is selected based on Frame Format and MCS
  frameFormat : Inport
  MCS : Inport  Port=2
  Constant : Constant  Value=true  SampleTime=1/inputSamplingRate
  Constant1 : Constant  Value=0  OutDataTypeStr=fixdt(0,5,0)  SampleTime=1/inputSamplingRate
  Constant11 : Constant  Value=4  OutDataTypeStr=fixdt(0,5,0)  SampleTime=1/inputSamplingRate
  Constant12 : Constant  Value=5  OutDataTypeStr=fixdt(0,5,0)  SampleTime=1/inputSamplingRate
  Constant13 : Constant  Value=6  OutDataTypeStr=fixdt(0,5,0)  SampleTime=1/inputSamplingRate
  Constant14 : Constant  Value=7  OutDataTypeStr=fixdt(0,5,0)  SampleTime=1/inputSamplingRate
  Constant15 : Constant  Value=11  OutDataTypeStr=fixdt(0,5,0)  SampleTime=1/inputSamplingRate
  Constant16 : Constant  Value=12  OutDataTypeStr=fixdt(0,5,0)  SampleTime=1/inputSamplingRate
  Constant17 : Constant  Value=13  OutDataTypeStr=fixdt(0,5,0)  SampleTime=1/inputSamplingRate
  Constant18 : Constant  Value=14  OutDataTypeStr=fixdt(0,5,0)  SampleTime=1/inputSamplingRate
  Constant19 : Constant  Value=15  OutDataTypeStr=fixdt(0,5,0)  SampleTime=1/inputSamplingRate
  Constant2 : Constant  OutDataTypeStr=fixdt(0,5,0)  SampleTime=1/inputSamplingRate
  Constant3 : Constant  Value=2  OutDataTypeStr=fixdt(0,5,0)  SampleTime=1/inputSamplingRate
  Constant4 : Constant  Value=3  OutDataTypeStr=fixdt(0,5,0)  SampleTime=1/inputSamplingRate
  Constant5 : Constant  Value=8  OutDataTypeStr=fixdt(0,5,0)  SampleTime=1/inputSamplingRate
  Constant6 : Constant  Value=9  OutDataTypeStr=fixdt(0,5,0)  SampleTime=1/inputSamplingRate
  Constant7 : Constant  Value=10  OutDataTypeStr=fixdt(0,5,0)  SampleTime=1/inputSamplingRate
  Delay : Delay
  Multiport Switch : MultiPortSwitch  DataPortOrder=Zero-based contiguous  Inputs=8  zeroidx=on  SaturateOnIntegerOverflow=off  InputSameDT=off
  Multiport Switch1 : MultiPortSwitch  Inputs=2  DataPortIndices={0,1,2,3,8,9,10,16,17,18}  SaturateOnIntegerOverflow=off  InputSameDT=off
  Multiport Switch2 : MultiPortSwitch  DataPortOrder=Zero-based contiguous  Inputs=8  DataPortIndices={8,9,10}  zeroidx=on  SaturateOnIntegerOverflow=off  InputSameDT=off
  Tx_LUT_Selection : Subsystem
  txData : Outport
  txValid : Outport  Port=2
  wires:
  Multiport Switch1/1 -> Tx_LUT_Selection/1(LUTSelect)
  Constant1/1 -> Multiport Switch/2
  Constant/1 -> Delay/1
  Constant3/1 -> Multiport Switch/4
  Constant5/1 -> Multiport Switch2/2
  Constant4/1 -> Multiport Switch/5
  Constant6/1 -> Multiport Switch2/3
  Multiport Switch/1 -> Multiport Switch1/2
  MCS/1 -> Multiport Switch/1, Multiport Switch2/1
  Constant2/1 -> Multiport Switch/3
  Constant7/1 -> Multiport Switch2/4
  Tx_LUT_Selection/1(txData) -> txData/1
  frameFormat/1 -> Multiport Switch1/1
  Multiport Switch2/1 -> Multiport Switch1/3
  Delay/1 -> txValid/1
  Constant11/1 -> Multiport Switch/6
  Constant12/1 -> Multiport Switch/7
  Constant13/1 -> Multiport Switch/8
  Constant14/1 -> Multiport Switch/9
  Constant15/1 -> Multiport Switch2/5
  Constant16/1 -> Multiport Switch2/6
  Constant17/1 -> Multiport Switch2/7
  Constant18/1 -> Multiport Switch2/8
  Constant19/1 -> Multiport Switch2/9
